simulink model "A2_Testing_final"  (R2024a)
settings: Solver=FixedStepAuto  StartTime=0.0  StopTime=10.0  FixedStep=1e-3  RelTol=1e-3  EnableMultiTasking=on
undefined symbols (not defined in the file): A0, A1, D0, D1, D10, D11, D12, D13, D2, D3, D4, D5, D6, D7, D8, D9, PTA0, PTA1, PTA2, PTB2, PTB23, PTB3, PTB9, PTC16, PTC17, PTC2, PTC3, PTC4, PTD0, PTD1, PTD2, PTD3
libraries: frdmk64flib x21, etargetslib x2
settings Model: ExtModeTrigDuration=5  Creator=haani  LastModifiedBy=hmz04
settings OptimizationCC: EnhancedBackFolding=on  PassReuseOutputArgsAs=Individual arguments  ZeroExternalMemoryAtStartup=off  ZeroInternalMemoryAtStartup=off  MaxStackSize=64  OptimizeBlockOrder=speed  DifferentSizesBufferReuse=on  OptimizationCustomize=off  EfficientTunableParamExpr=on
settings DebuggingCC: ParameterTunabilityLossMsg=error
settings HardwareCC: ProdBitPerPointer=32  ProdBitPerSizeT=32  ProdBitPerPtrDiffT=32  ProdLargestAtomicInteger=Long  ProdLargestAtomicFloat=Double  ProdWordSize=32  ProdHWDeviceType=ARM Compatible->ARM Cortex
settings SFSimCC: MATLABDynamicMemAlloc=off
settings RTWCC: Description=Embedded Coder  SystemTargetFile=ert.tlc  HardwareBoard=NXP FRDM-K64F  TLCOptions="-aInlineSetEventsForThisBaseRateFcn=TLC_FALSE -aSuppressMultiTaskScheduler=TLC_FALSE  -aRateBasedStepFcn=0"  TemplateMakefile=ert_default_tmf  Toolchain=GNU Tools for ARM Embedded Processors
settings CodeAppCC: ForceParamTrailComments=on  IgnoreCustomStorageClasses=off  OperatorAnnotations=on  SimulinkDataObjDesc=on  SFDataObjDesc=on  InsertBlockDesc=on
settings ERTTargetCC: ExtModeTransport=4  ExtModeMexFile=sendToCommService

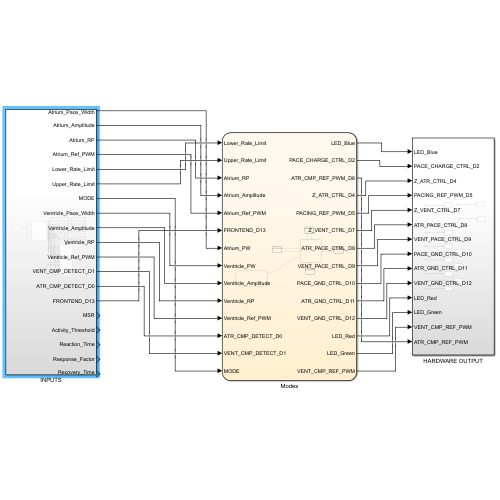
[thumbnail: Simulink's stored preview of the top-level diagram]
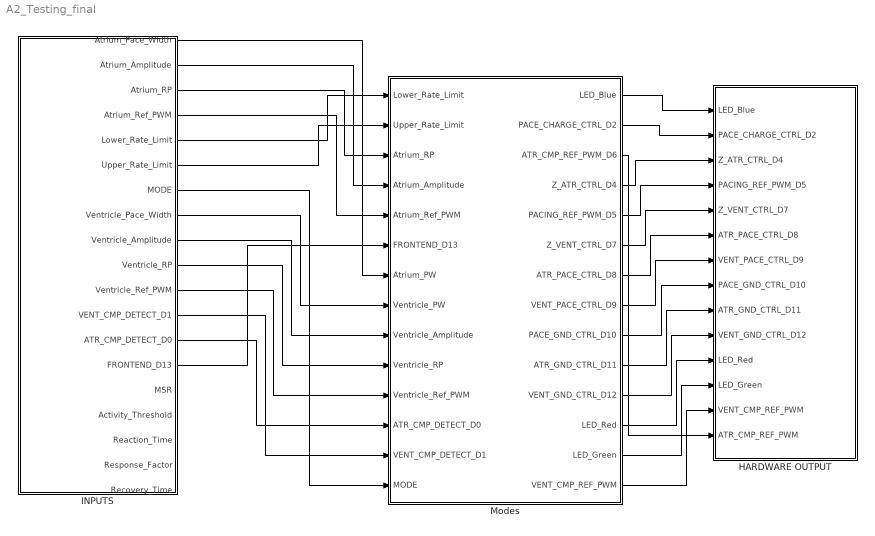
== system A2_Testing_final ==
  HARDWARE OUTPUT : Subsystem
  INPUTS : Subsystem
  Modes : Stateflow chart  TreatAsAtomicUnit=on
  wires:
  Modes/1(LED_Blue) -> HARDWARE OUTPUT/1(LED_Blue)
  Modes/2(PACE_CHARGE_CTRL_D2) -> HARDWARE OUTPUT/2(PACE_CHARGE_CTRL_D2)
  Modes/4(Z_ATR_CTRL_D4) -> HARDWARE OUTPUT/3(Z_ATR_CTRL_D4)
  Modes/5(PACING_REF_PWM_D5) -> HARDWARE OUTPUT/4(PACING_REF_PWM_D5)
  Modes/6(Z_VENT_CTRL_D7) -> HARDWARE OUTPUT/5(Z_VENT_CTRL_D7)
  Modes/7(ATR_PACE_CTRL_D8) -> HARDWARE OUTPUT/6(ATR_PACE_CTRL_D8)
  Modes/8(VENT_PACE_CTRL_D9) -> HARDWARE OUTPUT/7(VENT_PACE_CTRL_D9)
  Modes/9(PACE_GND_CTRL_D10) -> HARDWARE OUTPUT/8(PACE_GND_CTRL_D10)
  Modes/10(ATR_GND_CTRL_D11) -> HARDWARE OUTPUT/9(ATR_GND_CTRL_D11)
  Modes/11(VENT_GND_CTRL_D12) -> HARDWARE OUTPUT/10(VENT_GND_CTRL_D12)
  INPUTS/5(Lower_Rate_Limit) -> Modes/1(Lower_Rate_Limit)
  INPUTS/6(Upper_Rate_Limit) -> Modes/2(Upper_Rate_Limit)
  INPUTS/1(Atrium_Pace_Width) -> Modes/7(Atrium_PW)
  INPUTS/2(Atrium_Amplitude) -> Modes/4(Atrium_Amplitude)
  INPUTS/3(Atrium_RP) -> Modes/3(Atrium_RP)
  INPUTS/4(Atrium_Ref_PWM) -> Modes/5(Atrium_Ref_PWM)
  Modes/12(LED_Red) -> HARDWARE OUTPUT/11(LED_Red)
  Modes/13(LED_Green) -> HARDWARE OUTPUT/12(LED_Green)
  Modes/3(ATR_CMP_REF_PWM_D6) -> HARDWARE OUTPUT/14(ATR_CMP_REF_PWM)
  INPUTS/8(Ventricle_Pace_Width) -> Modes/8(Ventricle_PW)
  INPUTS/7(" MODE") -> Modes/14(MODE)
  INPUTS/9(Ventricle_Amplitude) -> Modes/9(Ventricle_Amplitude)
  INPUTS/10(Ventricle_RP) -> Modes/10(Ventricle_RP)
  INPUTS/11(Ventricle_Ref_PWM) -> Modes/11(Ventricle_Ref_PWM)
  Modes/14(VENT_CMP_REF_PWM) -> HARDWARE OUTPUT/13(VENT_CMP_REF_PWM)
  INPUTS/14(FRONTEND_D13) -> Modes/6(FRONTEND_D13)
  INPUTS/13(ATR_CMP_DETECT_D0) -> Modes/12(ATR_CMP_DETECT_D0)
  INPUTS/12(VENT_CMP_DETECT_D1) -> Modes/13(VENT_CMP_DETECT_D1)

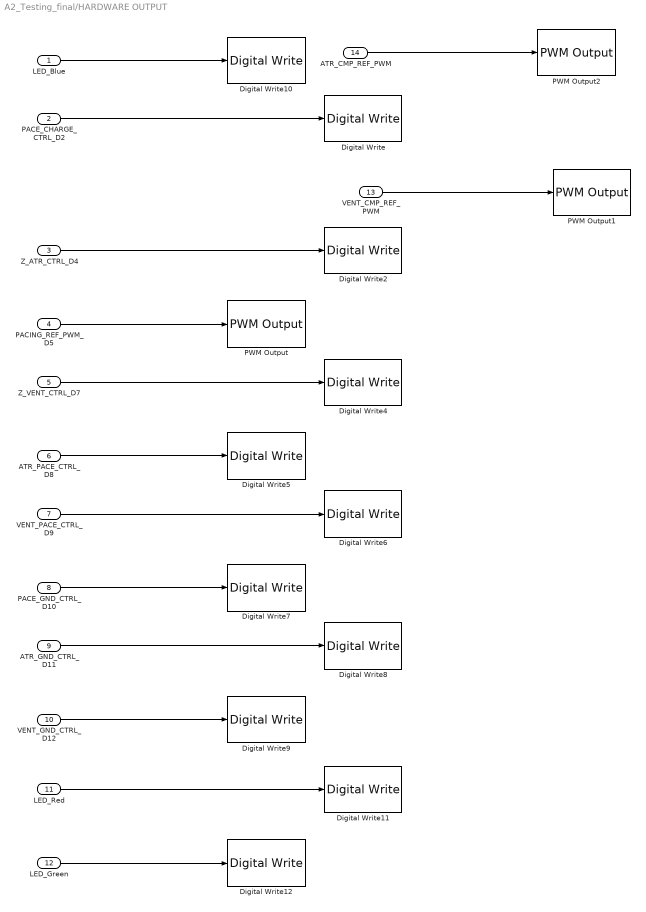
== system A2_Testing_final/HARDWARE OUTPUT ==
  LED_Blue : Inport
  PACE_CHARGE_CTRL_D2 : Inport  Port=2
  Z_ATR_CTRL_D4 : Inport  Port=3
  PACING_REF_PWM_D5 : Inport  Port=4
  Z_VENT_CTRL_D7 : Inport  Port=5
  ATR_PACE_CTRL_D8 : Inport  Port=6
  VENT_PACE_CTRL_D9 : Inport  Port=7
  PACE_GND_CTRL_D10 : Inport  Port=8
  ATR_GND_CTRL_D11 : Inport  Port=9
  VENT_GND_CTRL_D12 : Inport  Port=10
  LED_Red : Inport  Port=11
  LED_Green : Inport  Port=12
  VENT_CMP_REF_PWM : Inport  Port=13
  ATR_CMP_REF_PWM : Inport  Port=14
  Digital Write : frdmk64flib/Digital Write  Whichpin=PTB9 (D2)
  Digital Write10 : frdmk64flib/Digital Write  Whichpin=BLUE_LED
  Digital Write11 : frdmk64flib/Digital Write  Whichpin=RED_LED
  Digital Write12 : frdmk64flib/Digital Write  Whichpin=GREEN_LED
  Digital Write2 : frdmk64flib/Digital Write  Whichpin=PTB23 (D4)
  Digital Write4 : frdmk64flib/Digital Write  Whichpin=PTC3 (D7)
  Digital Write5 : frdmk64flib/Digital Write  Whichpin=PTA0 (D8)
  Digital Write6 : frdmk64flib/Digital Write  Whichpin=PTC4 (D9)
  Digital Write7 : frdmk64flib/Digital Write  Whichpin=PTD0 (D10)
  Digital Write8 : frdmk64flib/Digital Write  Whichpin=PTD2 (D11)
  Digital Write9 : frdmk64flib/Digital Write  Whichpin=PTD3 (D12)
  PWM Output : frdmk64flib/PWM Output  Whichpin=PTA2 (D5)  InitialFrequency=2000  InitialDutyCycle=0
  PWM Output1 : frdmk64flib/PWM Output  Whichpin=PTA1 (D3)  InitialFrequency=2000  InitialDutyCycle=0
  PWM Output2 : frdmk64flib/PWM Output  Whichpin=PTC2 (D6)  InitialFrequency=2000  InitialDutyCycle=0
  wires:
  LED_Blue/1 -> Digital Write10/1
  PACE_CHARGE_CTRL_D2/1 -> Digital Write/1
  Z_ATR_CTRL_D4/1 -> Digital Write2/1
  PACING_REF_PWM_D5/1 -> PWM Output/1
  Z_VENT_CTRL_D7/1 -> Digital Write4/1
  ATR_GND_CTRL_D11/1 -> Digital Write8/1
  PACE_GND_CTRL_D10/1 -> Digital Write7/1
  ATR_PACE_CTRL_D8/1 -> Digital Write5/1
  VENT_PACE_CTRL_D9/1 -> Digital Write6/1
  VENT_GND_CTRL_D12/1 -> Digital Write9/1
  LED_Green/1 -> Digital Write12/1
  LED_Red/1 -> Digital Write11/1
  VENT_CMP_REF_PWM/1 -> PWM Output1/1
  ATR_CMP_REF_PWM/1 -> PWM Output2/1

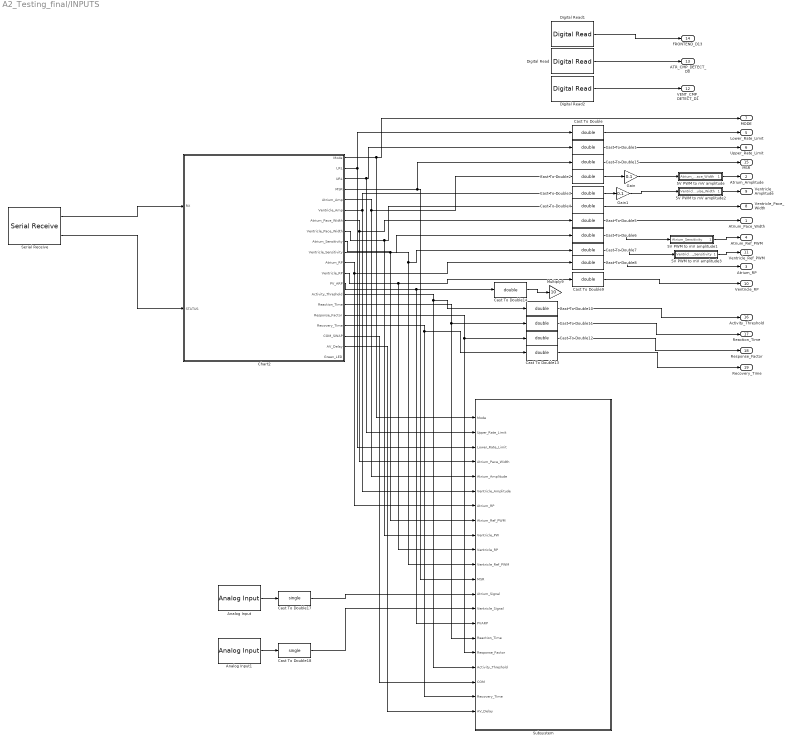
== system A2_Testing_final/INPUTS ==
  " 5V PWM to mV amplitude1" : Subsystem
  5V PWM to mV amplitude : Subsystem
  5V PWM to mV amplitude2 : Subsystem
  5V PWM to mV amplitude3 : Subsystem
  Analog Input : frdmk64flib/Analog Input  Whichpin=PTB2 (A0)  SampleTime=-1
  Analog Input1 : frdmk64flib/Analog Input  Whichpin=PTB3 (A1)  SampleTime=-1
  Cast To Double{,1..15} (16 alike) : DataTypeConversion  OutDataTypeStr=double  SaturateOnIntegerOverflow=off  RndMeth=Floor
  Cast To Double17 : DataTypeConversion  OutDataTypeStr=single  SaturateOnIntegerOverflow=off  RndMeth=Floor
  Cast To Double18 : DataTypeConversion  OutDataTypeStr=single  SaturateOnIntegerOverflow=off  RndMeth=Floor
  Chart2 : Stateflow chart  TreatAsAtomicUnit=on
      settings: PortSchema="{\"entries\":[{\"content\":{\"sides\":[{\"content\":{\"connectorIds\":[\"In1\",\"In2\"]},\"type\":\"ConnectorPlacement.EquallySpacedRectSide\",\"uuid\":\"ffb3d753-dbd9-4cc9-b3f6-be85e99fedf4\"},{\"content\":{\"connectorIds\":[\"Out1\",\"Out2\",\"Out3\",\"Out4\",\"Out5\",\"Out6\",\"Out7\",\"Out8\",\"Out9\",\"Out10\",\"Out11\",\"Out12\",\"Out13\",\"Out14\",\"Out15\",\"Out16\",\"Out17\",\"Out20\",\"Out19\",\"Out18\"],\"side\":\"RIGHT\"},\"type\":\"ConnectorPlacement.EquallySpacedRectSide\",\"uuid\":\"d9281469-7b65-4fbb-b110-42e9dc9d143e\"},{\"content\":{\"side\":\"TOP\"},\"type\":\"ConnectorPlacement.EquallySpacedRectSide\",\"uuid\":\"c04fd83a-1ddb-447c-b8da-2c1ff021f229\"}]},\"type\":\"ConnectorPlacement.EquallySpacedConnector\",\"uuid\":\"b5cd29c2-8e65-48be-b85d-9c735eabd7c7\"}],\"packageUris\":[\"http://schema.mathworks.com/mf0/Connector/R2020b\"],\"version\":\"1.0\"}"
  Digital Read : frdmk64flib/Digital Read  Whichpin=PTC16 (D0)  SampleTime=-1
  Digital Read1 : frdmk64flib/Digital Read  Whichpin=PTD1 (D13)  SampleTime=-1
  Digital Read2 : frdmk64flib/Digital Read  Whichpin=PTC17 (D1)  SampleTime=-1
  Gain : Gain  Gain=0.1
  Gain1 : Gain  Gain=0.1
  Multiply9 : Gain  Gain=10
  Serial Receive : frdmk64flib/Serial Receive  SCIModule=0  Baudrate=uint32(9600)  Parity=None  StopBits=1  HardwareFlowControl=None  ByteOrder=LittleEndian  DataType=uint8  DataLength=20  BlockingMode=off  OutputStatus=on  SampleTime=-1
  Subsystem : Subsystem
  Atrium_Pace_Width : Outport
  Atrium_Amplitude : Outport  Port=2
  Atrium_RP : Outport  Port=3
  Atrium_Ref_PWM : Outport  Port=4
  Lower_Rate_Limit : Outport  Port=5
  Upper_Rate_Limit : Outport  Port=6
  " MODE" : Outport  Port=7
  Ventricle_Pace_Width : Outport  Port=8
  Ventricle_Amplitude : Outport  Port=9
  Ventricle_RP : Outport  Port=10
  Ventricle_Ref_PWM : Outport  Port=11
  VENT_CMP_DETECT_D1 : Outport  Port=12
  ATR_CMP_DETECT_D0 : Outport  Port=13
  FRONTEND_D13 : Outport  Port=14
  MSR : Outport  Port=15
  Activity_Threshold : Outport  Port=16
  Reaction_Time : Outport  Port=17
  Response_Factor : Outport  Port=18
  Recovery_Time : Outport  Port=19
  wires:
  Digital Read/1 -> ATR_CMP_DETECT_D0/1
  Digital Read2/1 -> VENT_CMP_DETECT_D1/1
  Digital Read1/1 -> FRONTEND_D13/1
  5V PWM to mV amplitude/1(" ") -> Atrium_Amplitude/1
  " 5V PWM to mV amplitude1"/1(" ") -> Atrium_Ref_PWM/1
  5V PWM to mV amplitude2/1(" ") -> Ventricle_Amplitude/1
  5V PWM to mV amplitude3/1(" ") -> Ventricle_Ref_PWM/1
  Chart2/3(URL) -> Cast To Double1/1, Subsystem/2(Upper_Rate_Limit)
  Chart2/1(Mode) -> " MODE"/1, Subsystem/1(Mode)
  Chart2/2(LRL) -> Cast To Double/1, Subsystem/3(Lower_Rate_Limit)
  Chart2/4(MSR) -> Cast To Double15/1, Subsystem/12(MSR)
  Chart2/5(Atrium_Amp) -> Cast To Double2/1, Subsystem/5(Atrium_Amplitude)
  Chart2/6(Ventricle_Amp) -> Subsystem/6(Ventricle_Amplitude), Cast To Double3/1
  Chart2/8(Ventricle_Pace_Width) -> Cast To Double4/1, Subsystem/9(Ventricle_PW)
  Chart2/7(Atrium_Pace_Width) -> Cast To Double5/1, Subsystem/4(Atrium_Pace_Width)
  Chart2/9(Atrium_Sensitivity) -> Cast To Double6/1, Subsystem/8(Atrium_Ref_PWM)
  Chart2/10(Ventricle_Sensitivity) -> Cast To Double7/1, Subsystem/11(Ventricle_Ref_PWM)
  Chart2/11(Atrium_RP) -> Cast To Double8/1, Subsystem/7(Atrium_RP)
  Chart2/12(Ventricle_RP) -> Subsystem/10(Ventricle_RP), Cast To Double9/1
  Chart2/14(Activity_Threshold) -> Cast To Double10/1, Subsystem/18(Activity_Threshold)
  Chart2/15(Reaction_Time) -> Cast To Double11/1, Subsystem/16(Reaction_Time)
  Chart2/16(Response_Factor) -> Cast To Double12/1, Subsystem/17(Response_Factor)
  Chart2/17(Recovery_Time) -> Cast To Double13/1, Subsystem/20(Recovery_Time)
  Serial Receive/2 -> Chart2/2(STATUS)
  Chart2/20(COM_SWAP) -> Subsystem/19(COM)
  Chart2/19(AV_Delay) -> Subsystem/21(AV_Delay)
  Analog Input1/1 -> Cast To Double18/1
  Analog Input/1 -> Cast To Double17/1
  Cast To Double17/1 -> Subsystem/13(Atrium_Signal)
  Cast To Double18/1 -> Subsystem/14(Ventricle_Signal)
  Cast To Double/1 -> Lower_Rate_Limit/1
  Cast To Double1/1 -> Upper_Rate_Limit/1
  Cast To Double2/1 -> Gain/1
  Cast To Double3/1 -> Gain1/1
  Cast To Double4/1 -> Ventricle_Pace_Width/1
  Cast To Double5/1 -> Atrium_Pace_Width/1
  Cast To Double6/1 -> " 5V PWM to mV amplitude1"/1(Atrium_Sensitivity)
  Cast To Double7/1 -> 5V PWM to mV amplitude3/1(Ventricle_Sensitivity)
  Cast To Double8/1 -> Atrium_RP/1
  Cast To Double9/1 -> Ventricle_RP/1
  Cast To Double10/1 -> Activity_Threshold/1
  Cast To Double11/1 -> Reaction_Time/1
  Cast To Double12/1 -> Response_Factor/1
  Cast To Double13/1 -> Recovery_Time/1
  Chart2/13(PV_ARP) -> Subsystem/15(PVARP), Cast To Double14/1
  Cast To Double14/1 -> Multiply9/1
  Gain/1 -> 5V PWM to mV amplitude/1(Atrium_Pace_Width)
  Gain1/1 -> 5V PWM to mV amplitude2/1(Ventricle_Pulse_Width)
  Cast To Double15/1 -> MSR/1
  Serial Receive/1 -> Chart2/1(RX)

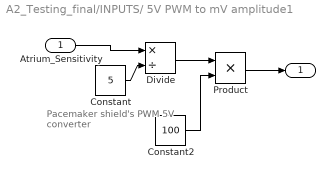
== system A2_Testing_final/INPUTS/ 5V PWM to mV amplitude1 ==
  note: Pacemaker shield's PWM 5V converter
  Atrium_Sensitivity : Inport
  Constant : Constant  Value=5
  Constant2 : Constant  Value=100
  Divide : Product  Inputs=*/
  Product : Product
  " " : Outport
  wires:
  Divide/1 -> Product/1
  Constant2/1 -> Product/2
  Constant/1 -> Divide/2
  Atrium_Sensitivity/1 -> Divide/1
  Product/1 -> " "/1

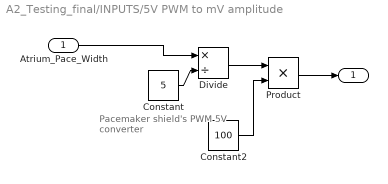
== system A2_Testing_final/INPUTS/5V PWM to mV amplitude ==
  note: Pacemaker shield's PWM 5V converter
  Atrium_Pace_Width : Inport
  Constant : Constant  Value=5
  Constant2 : Constant  Value=100
  Divide : Product  Inputs=*/
  Product : Product
  " " : Outport
  wires:
  Divide/1 -> Product/1
  Constant2/1 -> Product/2
  Constant/1 -> Divide/2
  Atrium_Pace_Width/1 -> Divide/1
  Product/1 -> " "/1

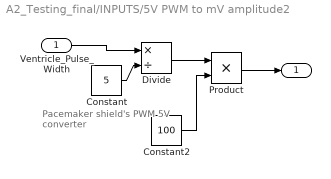
== system A2_Testing_final/INPUTS/5V PWM to mV amplitude2 ==
  note: Pacemaker shield's PWM 5V converter
  Ventricle_Pulse_Width : Inport
  Constant : Constant  Value=5
  Constant2 : Constant  Value=100
  Divide : Product  Inputs=*/
  Product : Product
  " " : Outport
  wires:
  Divide/1 -> Product/1
  Constant2/1 -> Product/2
  Constant/1 -> Divide/2
  Ventricle_Pulse_Width/1 -> Divide/1
  Product/1 -> " "/1

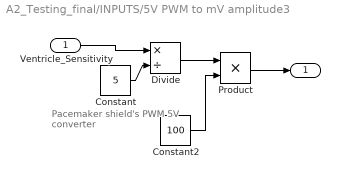
== system A2_Testing_final/INPUTS/5V PWM to mV amplitude3 ==
  note: Pacemaker shield's PWM 5V converter
  Ventricle_Sensitivity : Inport
  Constant : Constant  Value=5
  Constant2 : Constant  Value=100
  Divide : Product  Inputs=*/
  Product : Product
  " " : Outport
  wires:
  Divide/1 -> Product/1
  Constant2/1 -> Product/2
  Constant/1 -> Divide/2
  Ventricle_Sensitivity/1 -> Divide/1
  Product/1 -> " "/1

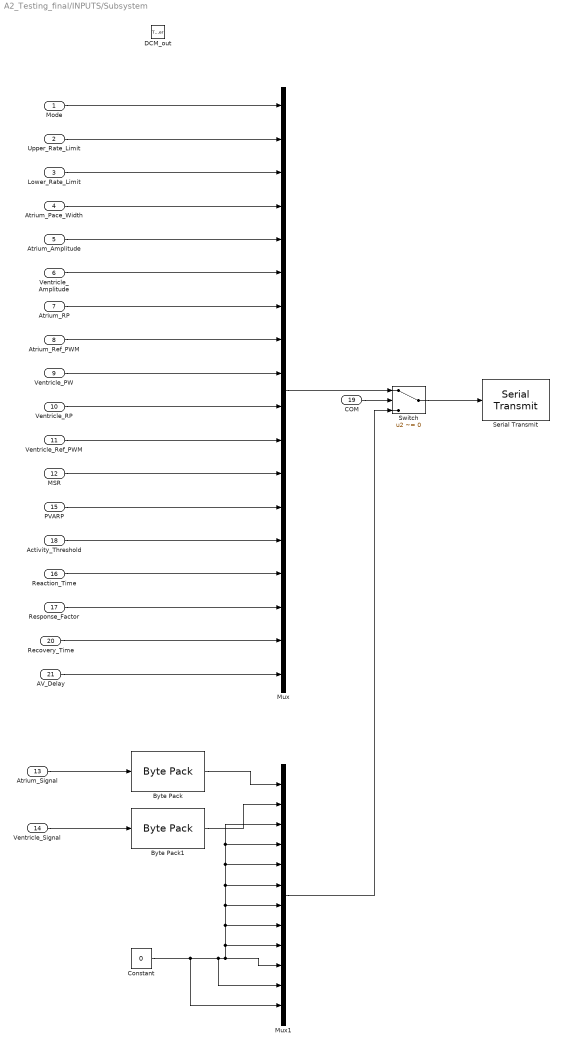
== system A2_Testing_final/INPUTS/Subsystem ==
  Mode : Inport
  Upper_Rate_Limit : Inport  Port=2
  Lower_Rate_Limit : Inport  Port=3
  Atrium_Pace_Width : Inport  Port=4
  Atrium_Amplitude : Inport  Port=5
  Ventricle_Amplitude : Inport  Port=6
  Atrium_RP : Inport  Port=7
  Atrium_Ref_PWM : Inport  Port=8
  Ventricle_PW : Inport  Port=9
  Ventricle_RP : Inport  Port=10
  Ventricle_Ref_PWM : Inport  Port=11
  MSR : Inport  Port=12
  Atrium_Signal : Inport  Port=13
  Ventricle_Signal : Inport  Port=14
  PVARP : Inport  Port=15
  Reaction_Time : Inport  Port=16
  Response_Factor : Inport  Port=17
  Activity_Threshold : Inport  Port=18
  COM : Inport  Port=19
  Recovery_Time : Inport  Port=20
  AV_Delay : Inport  Port=21
  DCM_out : TriggerPort  TriggerType=function-call  IsSimulinkFunction=on  FunctionName=DCM_out  VariantControl=(inherit)
  Byte Pack : etargetslib/Byte Pack  datatypes={'single'}  byteAlign=1
  Byte Pack1 : etargetslib/Byte Pack  datatypes={'single'}  byteAlign=1
  Constant : Constant  Value=0  OutDataTypeStr=uint8
  Mux : Mux  Inputs=18
  Mux1 : Mux  Inputs=12
  Serial Transmit : frdmk64flib/Serial Transmit  SCIModule=0  Baudrate=uint32(9600)  Parity=None  StopBits=1  HardwareFlowControl=None  ByteOrder=LittleEndian  BlockingMode=on  OutputStatus=off
  Switch : Switch  Criteria=u2 ~= 0  SaturateOnIntegerOverflow=off  InputSameDT=off
  wires:
  Mode/1 -> Mux/1
  Upper_Rate_Limit/1 -> Mux/2
  Lower_Rate_Limit/1 -> Mux/3
  Atrium_Pace_Width/1 -> Mux/4
  Atrium_Amplitude/1 -> Mux/5
  Ventricle_Amplitude/1 -> Mux/6
  Atrium_RP/1 -> Mux/7
  Atrium_Ref_PWM/1 -> Mux/8
  Ventricle_PW/1 -> Mux/9
  Ventricle_RP/1 -> Mux/10
  Ventricle_Ref_PWM/1 -> Mux/11
  MSR/1 -> Mux/12
  PVARP/1 -> Mux/13
  Activity_Threshold/1 -> Mux/14
  Reaction_Time/1 -> Mux/15
  Response_Factor/1 -> Mux/16
  Recovery_Time/1 -> Mux/17
  COM/1 -> Switch/2
  Switch/1 -> Serial Transmit/1
  Ventricle_Signal/1 -> Byte Pack1/1
  Atrium_Signal/1 -> Byte Pack/1
  Byte Pack/1 -> Mux1/1
  Byte Pack1/1 -> Mux1/2
  Mux1/1 -> Switch/3
  Mux/1 -> Switch/1
  AV_Delay/1 -> Mux/18
  Constant/1 -> Mux1/12, Mux1/11, Mux1/10, Mux1/9, Mux1/8, Mux1/7, Mux1/4, Mux1/3, Mux1/5, Mux1/6

== stateflow chart A2_Testing_final/Modes ==
  state VVI
    state Refractory
      entry:
      PACING_REF_PWM_D5 = 100*(Ventricle_Amplitude/5)
      PACE_CHARGE_CTRL_D2=1;
      PACE_GND_CTRL_D10=1;
      VENT_PACE_CTRL_D9=0;
      Z_ATR_CTRL_D4=0;
      Z_VENT_CTRL_D7=0;
      ATR_PACE_CTRL_D8=0;
      ATR_GND_CTRL_D11=0;
      VENT_GND_CTRL_D12=1;
      VENT_CMP_REF_PWM= Ventricle_Ref_PWM;
      %Visual Signal
      LED_Blue=0;
      Period=60000/(Lower_Rate_Limit)
    state Pace
      entry:
      PACING_REF_PWM_D5=0
      PACE_CHARGE_CTRL_D2=0;
      PACE_GND_CTRL_D10=1;
      ATR_PACE_CTRL_D8=0;
      ATR_GND_CTRL_D11=0;
      Z_ATR_CTRL_D4=0;
      Z_VENT_CTRL_D7=0;
      VENT_GND_CTRL_D12=0;
      VENT_PACE_CTRL_D9=1;
      %Visual Signal
      LED_Blue=1;
      LED_Green=0;
    state Sense
      entry:
      LED_Green = 1;
    VVI.Pace -> VVI.Refractory : [after(Ventricle_PW,msec)]
    (default) -> VVI.Refractory
    VVI.Refractory -> VVI.Sense : [after(Ventricle_RP,msec)]
    VVI.Sense -> VVI.Pace [order 1] : [after(Period-Ventricle_RP-Ventricle_PW,msec)]
    VVI.Sense -> VVI.Refractory [order 2] : [VENT_CMP_DETECT_D1 == 1]
  state Mode
    %Reset everything
    entry:
    LED_Red  = 0;
    ATR_PACE_CTRL_D8 = 0;
    ATR_GND_CTRL_D11 = 0;
    VENT_GND_CTRL_D12 = 0;
    VENT_PACE_CTRL_D9 = 0;
    Z_ATR_CTRL_D4 = 0;
    Z_VENT_CTRL_D7 = 0;
    ATR_CMP_REF_PWM_D6 = 0;
    VENT_CMP_REF_PWM= 0;
    PACE_GND_CTRL_D10 = 0;
    PACE_CHARGE_CTRL_D2 = 0;
  state VOO
    state ChargeDischarge
      entry:
      %DISCHARGE C21 (resets everything)
      PACE_GND_CTRL_D10 = 1;
      ATR_GND_CTRL_D11 = 0;
      VENT_GND_CTRL_D12 = 1;
      VENT_PACE_CTRL_D9 = 0;
      ATR_PACE_CTRL_D8 = 0;
      Z_ATR_CTRL_D4 = 0;
      Z_VENT_CTRL_D7 = 0;
      %CHARGE C22 (prepare for next pulse)
      PACE_CHARGE_CTRL_D2=1;
      PACING_REF_PWM_D5 = Ventricle_Amplitude;
      %VISUAL SIGNAL
      LED_Blue = 0;
      %TIMING
      STANDBY_PERIOD = 30000/(Lower_Rate_Limit);
    state Pace1
      entry:
      %PROPER GND + TRIGGER PACE
      PACE_GND_CTRL_D10 = 1;
      ATR_GND_CTRL_D11 = 0;
      VENT_GND_CTRL_D12 = 0;
      VENT_PACE_CTRL_D9 = 1;
      ATR_PACE_CTRL_D8 = 0;
      Z_ATR_CTRL_D4 = 0;
      Z_VENT_CTRL_D7 = 0;
      PACE_CHARGE_CTRL_D2=0;
      PACING_REF_PWM_D5 = 0;
      %VISUAL SIGNAL
      LED_Blue = 1;
    (default) -> VOO.ChargeDischarge
    Pace1 -> VOO.ChargeDischarge : [after(Ventricle_PW,msec)]
    VOO.ChargeDischarge -> Pace1 : [after(STANDBY_PERIOD,msec)]
  state AAI
    state Pace
      entry:
      PACING_REF_PWM_D5=0
      PACE_CHARGE_CTRL_D2=0;
      PACE_GND_CTRL_D10=1;
      ATR_PACE_CTRL_D8=1;
      ATR_GND_CTRL_D11=0;
      Z_ATR_CTRL_D4=0;
      Z_VENT_CTRL_D7=0;
      VENT_GND_CTRL_D12=0;
      VENT_PACE_CTRL_D9=0;
      %Visual Signal
      LED_Blue=1;
      LED_Green = 0;
    state Refractory
      entry:
      PACING_REF_PWM_D5 = 100*(Atrium_Amplitude/5)
      PACE_CHARGE_CTRL_D2=1;
      PACE_GND_CTRL_D10=1;
      VENT_PACE_CTRL_D9=0;
      Z_ATR_CTRL_D4=0;
      Z_VENT_CTRL_D7=0;
      ATR_PACE_CTRL_D8=0;
      ATR_GND_CTRL_D11=1;
      VENT_GND_CTRL_D12=0;
      ATR_CMP_REF_PWM_D6= Atrium_Ref_PWM;
      %Visual Signal
      LED_Blue=0;
      Period=60000/(Lower_Rate_Limit)
    state Sense
      entry:
      LED_Green = 1;
    AAI.Pace -> AAI.Refractory : [after(Atrium_PW,msec)]
    (default) -> AAI.Refractory
    AAI.Refractory -> AAI.Sense : [after(Atrium_RP,msec)]
    AAI.Sense -> AAI.Pace [order 1] : [after(Period-Atrium_RP-Atrium_PW,msec)]
    AAI.Sense -> AAI.Refractory [order 2] : [ATR_CMP_DETECT_D0 == 1]
  state AOO
    state ChargeDischarge
      entry:
      %DISCHARGE C21 (resets everything)
      PACE_GND_CTRL_D10 = 1;
      ATR_GND_CTRL_D11 = 1;
      VENT_GND_CTRL_D12 = 0;
      VENT_PACE_CTRL_D9 = 0;
      ATR_PACE_CTRL_D8 = 0;
      Z_ATR_CTRL_D4 = 0;
      Z_VENT_CTRL_D7 = 0;
      %CHARGE C22 (prepare for next pulse)
      PACE_CHARGE_CTRL_D2=1;
      PACING_REF_PWM_D5 = Atrium_Amplitude;
      %VISUAL SIGNAL
      LED_Blue = 0;
      %TIMING
      STANDBY_PERIOD = 30000/(Lower_Rate_Limit);
    state Pace
      entry:
      %PROPER GND + TRIGGER PACE
      PACE_GND_CTRL_D10 = 1;
      ATR_GND_CTRL_D11 = 0;
      VENT_GND_CTRL_D12 = 0;
      VENT_PACE_CTRL_D9 = 0;
      ATR_PACE_CTRL_D8 = 1;
      Z_ATR_CTRL_D4 = 0;
      Z_VENT_CTRL_D7 = 0;
      PACE_CHARGE_CTRL_D2=0;
      PACING_REF_PWM_D5 = 0;
      %VISUAL SIGNAL
      LED_Blue = 1;
    (default) -> AOO.ChargeDischarge
    AOO.Pace -> AOO.ChargeDischarge : [after(Atrium_PW,msec)]
    AOO.ChargeDischarge -> AOO.Pace : [after(STANDBY_PERIOD,msec)]
  state Safety
    %LED turns red if any of the user input values are unsafe
    entry:
    LED_Red = 1;
  Mode -> VVI [order 4] : [MODE==3]
  VVI -> Mode : [MODE~=3]
  Mode -> VOO [order 2] : [MODE==2]
  AAI -> Mode : [MODE~=4]
  VOO -> Mode : [MODE~=2]
  Mode -> AAI [order 3] : [MODE==4]
  Safety -> Mode
  Mode -> AOO [order 1] : [MODE==1]
  AOO -> Mode : [MODE~=1]
  (default) -> Safety
  data: LED_Blue output; PACE_CHARGE_CTRL_D2 output; ATR_CMP_REF_PWM_D6 output; Z_ATR_CTRL_D4 output; PACING_REF_PWM_D5 output; Z_VENT_CTRL_D7 output; ATR_PACE_CTRL_D8 output; VENT_PACE_CTRL_D9 output; PACE_GND_CTRL_D10 output; ATR_GND_CTRL_D11 output; VENT_GND_CTRL_D12 output; Lower_Rate_Limit input; Upper_Rate_Limit input; Atrium_RP input; Atrium_Amplitude input; Atrium_Ref_PWM input; FRONTEND_D13 input; Atrium_PW input; Ventricle_PW input; Ventricle_Amplitude input; Ventricle_RP input; Ventricle_Ref_PWM input; ATR_CMP_DETECT_D0 input; VENT_CMP_DETECT_D1 input; LED_Red output; LED_Green output; Standby_Period local; MODE input; Period local; STANDBY_PERIOD local; VENT_CMP_REF_PWM output

== stateflow chart A2_Testing_final/INPUTS/Chart2 ==
  state Send_EGRAM
    entry:
    COM_SWAP=0;
    DCM_out(); %activate DCM_out subsystem
    Green_LED= 1;
    exit:
    COM_SWAP=1;
    Green_LED= 0 ;
  state Default_values
    %initalize all values
    entry:
    Mode=1;   %int unit8
    LRL=40;   %BPM uint8
    URL=180;   %BPM uint8
    MSR=120;   %BPM uint8
    AV_Delay=150;   %ms uint8
    Atrium_Amp=50   %mV single
    Ventricle_Amp=50;   %mV single
    Atrium_Pace_Width=1;   %ms single
    Ventricle_Pace_Width=1;   %ms single
    Atrium_Sensitivity=40;   %mV single
    Ventricle_Sensitivity=40;   %mV single
    Atrium_RP=25;   %ms uint16
    Ventricle_RP=32;   %ms uint16
    PV_ARP=32;   %ms uint16
    Activity_Threshold=4;   %int uint8
    Reaction_Time=30;   %s uint8
    Response_Factor=8   %int uint8
    Recovery_Time=5;   %min uint8
    Green_LED= 0; %sending to DCM_out
    COM_SWAP=1;
  state entry_RX
    %Take all initial values from DCM(RX)
    exit:
    MODE_IN = RX(1);
    LRL_IN = RX(2);
    URL_IN = RX(3);
    MSR_IN = RX(4);
    AVDELAY_IN = RX(5);
    ATRIUM_AMP_IN = RX(6); %divided by 10
    VENTRICLE_AMP_IN = RX(7); %divided by 10
    ATRIUM_PULSE_WIDTH_IN = RX(8);
    VENTRICLE_PULSE_WIDTH_IN = RX(9);
    ATRIUM_SENSITIVITY_IN = RX(10);
    VENTRICLE_SENSITIVITY_IN = RX(11);
    ATRIUM_RP_IN = RX(12);
    VENTRICLE_RP_IN = RX(13);
    PV_ARP_IN = RX(14);
    ACTIVITY_THRESHOLD_IN = RX(15);
    REACTION_TIME_IN = RX(16);
    RESPONSE_FACTOR_IN = RX(17);
    RECOVERY_TIME_IN = RX(18);
    SYNC_IN = RX(19);
    FUNCTION_IN = RX(20);
  state DCM_reentry
    entry:
    %Initialize variable to DCM input
    Mode= MODE_IN;
    LRL= LRL_IN;
    URL= URL_IN;
    MSR = MSR_IN;
    AV_Delay= AVDELAY_IN;
    Atrium_Amp= ATRIUM_AMP_IN;
    Ventricle_Amp=VENTRICLE_AMP_IN;
    Atrium_Pace_Width=ATRIUM_PULSE_WIDTH_IN;
    Ventricle_Pace_Width=VENTRICLE_PULSE_WIDTH_IN;
    Atrium_Sensitivity= ATRIUM_SENSITIVITY_IN;
    Ventricle_Sensitivity=VENTRICLE_SENSITIVITY_IN;
    Atrium_RP= ATRIUM_RP_IN;
    Ventricle_RP=VENTRICLE_RP_IN;
    PV_ARP= PV_ARP_IN;
    Activity_Threshold= ACTIVITY_THRESHOLD_IN;
    Reaction_Time= REACTION_TIME_IN;
    Response_Factor= RESPONSE_FACTOR_IN;
    Recovery_Time= RECOVERY_TIME_IN;
  state name
  state Wait
    entry:
  state Wait1
  state Return_Data
    entry:
    DCM_out(); %activate DCM_out subsystem
  Send_EGRAM -> entry_RX
  (default) -> Default_values
  Wait -> Send_EGRAM [order 3] : [FUNCTION_IN==56]
  entry_RX -> name : [STATUS==0]
  Wait -> DCM_reentry [order 1] : [FUNCTION_IN==85]
  name -> Wait : [SYNC_IN == 22]
  Wait -> Wait1 [order 2] : [FUNCTION_IN==34]
  Wait1 -> Return_Data : [after(20,msec)]
  DCM_reentry -> entry_RX
  Return_Data -> entry_RX
  Default_values -> entry_RX
  data: RX input; Mode output; FUNC local; SYNC local; STATUS input; LRL output; URL output; MSR output; Atrium_Amp output; Ventricle_Amp output; Atrium_Pace_Width output; Ventricle_Pace_Width output; Atrium_Sensitivity output; Ventricle_Sensitivity output; Atrium_RP output; Ventricle_RP output; PV_ARP output; LRLIN local; Activity_Threshold output; Reaction_Time output; Response_Factor output; Recovery_Time output; MSRIN local; URLIN local; AAmpIN local; AVDelayIN local; ARPIN local; APulseWidthIN local; ASensitivityIN local; ActivityThresholdIN local; MODEIN local; PVARPIN local; ReactionTimeIN local; RecoveryTimeIN local; ResponseFactorIN local; VAmpIN local; VPulseWidthIN local; VRPIN local; VSensitivityIN local; Green_LED output; AV_Delay output; COM_SWAP output; LRL_IN local; URL_IN local; SYNC_IN local; MODE_IN local; REACTION_TIME_IN local; ATRIUM_SENSITIVITY_IN local; ATRIUM_RP_IN local; RECOVERY_TIME_IN local; VENTRICLE_SENSITIVITY_IN local; ACTIVITY_THRESHOLD_IN local; FUNCTION_IN local; PVA_RP_IN local; ATRIUM_PULSE_WIDTH_IN local; RESPONSE_FACTOR_IN local; VENTRICLE_RP_IN local; VENTRICLE_AMP_IN local; VENTRICLE_PULSE_WIDTH_IN local; AVDELAY_IN local; ATRIUM_AMP_IN local; MSR_IN local; PV_ARP_IN local
